simulink model "Lab5_Lead"  (R2016a)
settings: Solver=VariableStepAuto  StartTime=0.0  StopTime=10.0  RelTol=1e-3
settings Model: Creator=jordan  LastModifiedBy=jordan

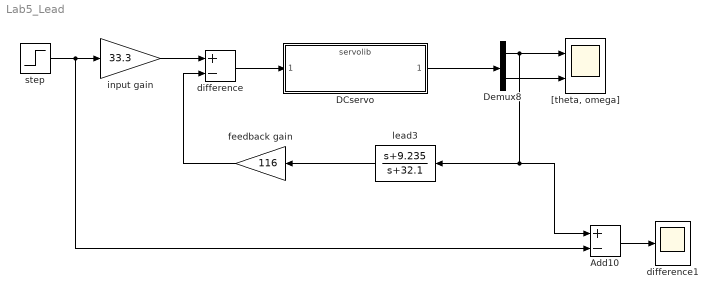
== system Lab5_Lead ==
  Add10 : Sum  Inputs=+-
  DCservo : ModelReference  ModelNameDialog=servolib.slx  SimulationMode=Normal  ModelReferenceVersion=1.68
  Demux8 : Demux  Outputs=2
  "[theta, omega]" : Scope  NumInputPorts=2
  difference : Sum  Inputs=+-
  difference1 : Scope
  feedback gain : Gain  Gain=116
  input gain : Gain  Gain=33.3
  lead3 : TransferFcn  Numerator=[1 9.235]  Denominator=[1 32.1]
  step : Step  SampleTime=0
  wires:
  Demux8/2 -> "[theta, omega]"/2
  step/1 -> Add10/2, input gain/1
  feedback gain/1 -> difference/2
  lead3/1 -> feedback gain/1
  input gain/1 -> difference/1
  Add10/1 -> difference1/1
  Demux8/1 -> Add10/1, lead3/1, "[theta, omega]"/1
  difference/1 -> DCservo/1
  DCservo/1 -> Demux8/1
